simulink model "avrdenemeson"  (R2023b)
settings: Solver=VariableStepAuto  StartTime=0.0  StopTime=10.0  RelTol=1e-3
settings Model: Creator=yasinsensoy  LastModifiedBy=yasinsensoy

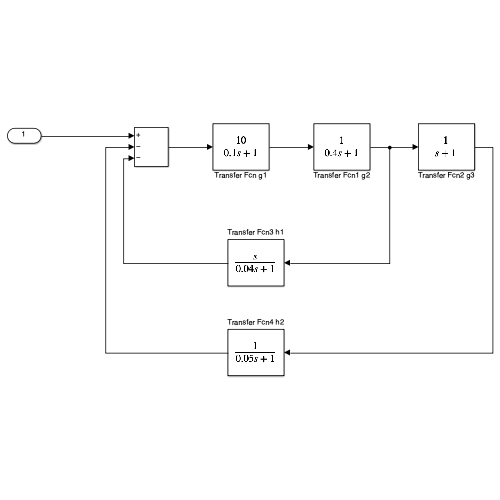
[thumbnail: Simulink's stored preview of the top-level diagram]
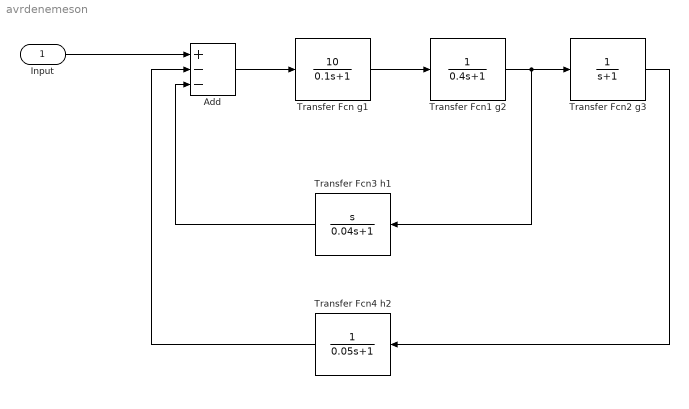
== system avrdenemeson ==
  Input : Inport
  Add : Sum  Inputs=+--
  Transfer Fcn g1 : TransferFcn  Numerator=[10]  Denominator=[0.1 1]
  Transfer Fcn1 g2 : TransferFcn  Denominator=[0.4 1]
  Transfer Fcn2 g3 : TransferFcn  Denominator=[1 1]
  Transfer Fcn3 h1 : TransferFcn  Numerator=[1 0]  Denominator=[0.04 1]
  Transfer Fcn4 h2 : TransferFcn  Denominator=[0.05 1]
  wires:
  Input/1 -> Add/1
  Add/1 -> Transfer Fcn g1/1
  Transfer Fcn g1/1 -> Transfer Fcn1 g2/1
  Transfer Fcn1 g2/1 -> Transfer Fcn3 h1/1, Transfer Fcn2 g3/1
  Transfer Fcn2 g3/1 -> Transfer Fcn4 h2/1
  Transfer Fcn3 h1/1 -> Add/3
  Transfer Fcn4 h2/1 -> Add/2
